simulink model "disturbances"  (R2026a)
settings: Solver=VariableStepAuto  StopTime=2000
settings Model: Creator=syane  LastModifiedBy=syane

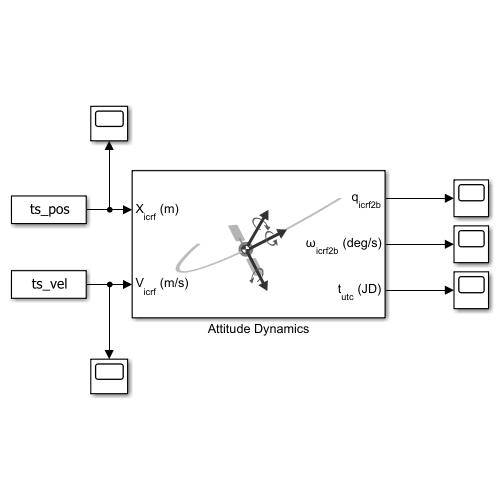
[thumbnail: Simulink's stored preview of the top-level diagram]
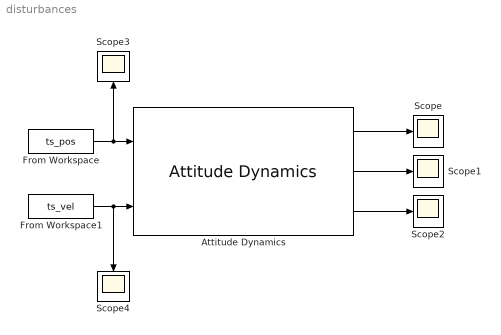
== system disturbances ==
  Attitude Dynamics : AttitudeDynamics  momentsIn=off
  From Workspace : FromWorkspace  VariableName=ts_pos
  From Workspace1 : FromWorkspace  VariableName=ts_vel
  Scope{,1..4} (5 alike) : Scope
      Scope settings: ActiveDisplayYMinimum=-1.1361470522677797  ActiveDisplayYMaximum=1.2373496724741977
      Scope1 settings: ActiveDisplayYMinimum=-1  ActiveDisplayYMaximum=1
      Scope2 settings: ActiveDisplayYMinimum=-1  ActiveDisplayYMaximum=1  DataLoggingVariableName=ScopeData2
      Scope3 settings: ActiveDisplayYMinimum=-53522.555780909941  ActiveDisplayYMaximum=53473.436359719686  DataLoggingVariableName=ScopeData3
      Scope4 settings: ActiveDisplayYMinimum=-1  ActiveDisplayYMaximum=1  DataLoggingVariableName=ScopeData4
  wires:
  From Workspace/1 -> Scope3/1, Attitude Dynamics/1
  From Workspace1/1 -> Scope4/1, Attitude Dynamics/2
  Attitude Dynamics/1 -> Scope/1
  Attitude Dynamics/2 -> Scope1/1
  Attitude Dynamics/3 -> Scope2/1
